simulink model "sl_closed_loop_1"  (R2019b)
settings: Solver=ode45  StartTime=0.0  StopTime=3  RelTol=1e-5  EnableMultiTasking=on
values from neighbouring files (symbols this model uses):
  A = zeros(4,4)    [closed_loop_1.m]    (also in closed_loop_2.m; open_loop.m)
  B = zeros(4,1)    [closed_loop_1.m]    (also in closed_loop_2.m; open_loop.m)
  C = eye(4)    [closed_loop_1.m]    (also in closed_loop_2.m = [1 0 0 0; open_loop.m = [1 0 0 0)
  D = zeros(4,1)    [closed_loop_1.m]    (also in closed_loop_2.m = [0; open_loop.m = zeros(2,1))
  K = K(1,:)    [closed_loop_1.m]    (also in closed_loop_2.m)
  x0 = [0  10*pi/180 0 0 ]    [closed_loop_1.m]    (also in closed_loop_2.m)
  x_d = [0.1 0 0 0]    [closed_loop_1.m]    (also in closed_loop_2.m)
settings Model: Creator=magudelo  LastModifiedBy=LouisDecloedt
settings DataIOCC: LimitDataPoints=on  SaveFormat=Array  SignalLoggingSaveFormat=ModelDataLogs  ReturnWorkspaceOutputs=off
settings OptimizationCC: ExpressionDepthLimit=2147483647  LifeSpan=inf
settings DebuggingCC: UnderspecifiedInitializationDetection=Classic  MergeDetectMultiDrivingBlocksExec=none  SolverPrmCheckMsg=warning  FcnCallInpInsideContextMsg=warning  AllowSymbolicDim=off  StateNameClashWarn=warning  SFUnexpectedBacktrackingDiag=warning  SFNoUnconditionalDefaultTransitionDiag=warning  SFExecutionAtInitializationDiag=none  ArithmeticOperatorsInVariantConditions=warning
settings HardwareCC: ProdBitPerPointer=32  ProdBitPerSizeT=32  ProdBitPerPtrDiffT=32  ProdLargestAtomicFloat=None  ProdIntDivRoundTo=Undefined  ProdEndianess=Unspecified  ProdWordSize=32  ProdHWDeviceType=32-bit Generic
settings ModelReferenceCC: PropagateSignalLabelsOutOfModel=off
settings SFSimCC: SimUseLocalCustomCode=off  CustomCodeUndefinedFunction=UseInterfaceOnly
settings RTWCC: RTWUseLocalCustomCode=off
settings CodeAppCC: StateflowObjectComments=on
settings GRTTargetCC: TargetLangStandard=C89/C90 (ANSI)  GeneratePreprocessorConditionals=Disable all  CombineOutputUpdateFcns=off  GRTInterface=on
settings ConfigComp: CovMetricSettings=dw  CovHtmlReporting=on  CovSaveCumulativeToWorkspaceVar=on  CovSaveSingleToWorkspaceVar=on  CovExternalEMLEnable=off

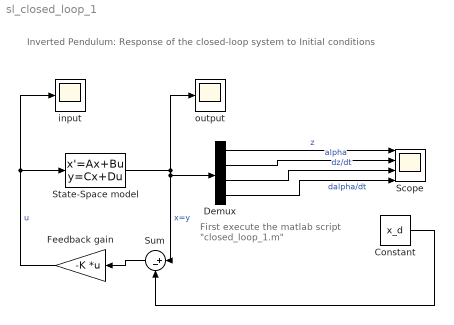
== system sl_closed_loop_1 ==
  note: First execute the matlab
      |  script "closed_loop_1.m"
  note: Inverted Pendulum: Response of the closed-loop system to Initial conditions
  Constant : Constant  Value=x_d
  Demux : Demux
  Feedback gain : Gain  Tag=Feedback gain  Description=f  Gain=-K  Multiplication=Matrix(K*u)
  Scope : Scope  NumInputPorts=4
  State-Space model : StateSpace  A=A  B=B  C=C  D=D  InitialCondition=x0
  Sum : Sum  Inputs=|+-
  input : Scope
  output : Scope
  wires:
  State-Space model/1 -> Sum/1, Demux/1, output/1  "x=y"
  Feedback gain/1 -> input/1, State-Space model/1  "u"
  Demux/1 -> Scope/1  "z"
  Demux/2 -> Scope/2  "alpha"
  Demux/3 -> Scope/3  "dz/dt"
  Demux/4 -> Scope/4  "dalpha/dt"
  Constant/1 -> Sum/2
  Sum/1 -> Feedback gain/1
